simulink model "MotorControllerSimulation"  (R2016b)
settings: Solver=FixedStepAuto  StartTime=0.0  StopTime=20  FixedStep=Ts.controller  RelTol=1e-3
undefined symbols (not defined in the file): motor, sys_d, Ts
libraries: simulink x1
settings Model: Creator=Wall  LastModifiedBy=Wall

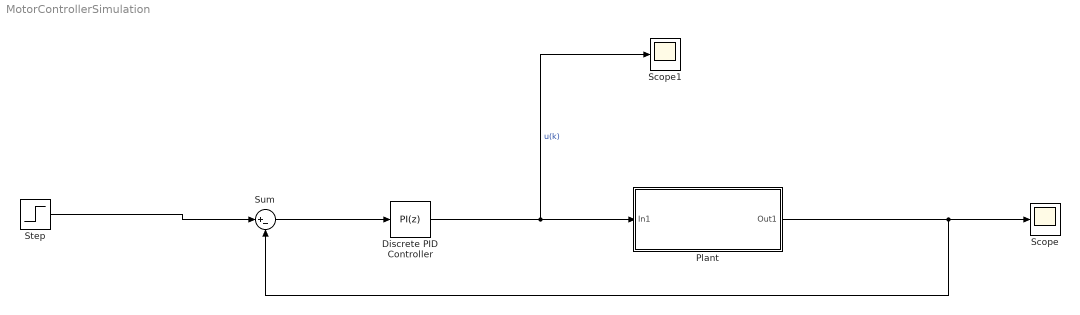
== system MotorControllerSimulation ==
  Discrete PID Controller : simulink/Continuous/PID Controller  Controller=PI  TimeDomain=Discrete-time  SampleTime=Ts.controller  IntegratorMethod=Forward Euler  FilterMethod=Forward Euler  Form=Parallel  UseFilter=off  ControllerParametersSource=internal  P=0.1  I=0.05  D=0  N=100  InitialConditionSource=internal  InitialConditionForIntegrator=0  InitialConditionForFilter=0  ExternalReset=none  LimitOutput=on  UpperSaturationLimit=motor.Imax  LowerSaturationLimit=-motor.Imax  LinearizeAsGain=off  AntiWindupMode=none  Kb=1  TrackingMode=off  Kt=1  PParamMin=[]  PParamMax=[]  IParamMin=[]  IParamMax=[]  DParamMin=[]  DParamMax=[]  NParamMin=[]  NParamMax=[]  KbParamMin=[]  KbParamMax=[]  KtParamMin=[]  KtParamMax=[]  POutMin=[]  POutMax=[]  IOutMin=[]  IOutMax=[]  DOutMin=[]  DOutMax=[]  NOutMin=[]  NOutMax=[]  KbOutMin=[]  KbOutMax=[]  KtOutMin=[]  KtOutMax=[]  IntegratorOutMin=[]  IntegratorOutMax=[]  FilterOutMin=[]  FilterOutMax=[]  SumOutMin=[]  SumOutMax=[]  SumI1OutMin=[]  SumI1OutMax=[]  SumI2OutMin=[]  SumI2OutMax=[]  SumI3OutMin=[]  SumI3OutMax=[]  SumDOutMin=[]  SumDOutMax=[]  SaturationOutMin=[]  SaturationOutMax=[]  IntegratorContinuousStateAttributes=''  IntegratorStateMustResolveToSignalObject=off  IntegratorRTWStateStorageClass=Auto  FilterContinuousStateAttributes=''  FilterStateMustResolveToSignalObject=off  FilterRTWStateStorageClass=Auto  DifferentiatorICPrevScaledInput=0  DifferentiatorOutMin=[]  DifferentiatorOutMax=[]
  Plant : Subsystem
  Scope : Scope
  Scope1 : Scope
  Step : Step  Time=2  After=200  SampleTime=Ts.controller
  Sum : Sum  Inputs=|+-
  wires:
  Discrete PID Controller/1 -> Plant/1(In1), Scope1/1  "u(k)"
  Sum/1 -> Discrete PID Controller/1
  Step/1 -> Sum/1
  Plant/1(Out1) -> Sum/2, Scope/1

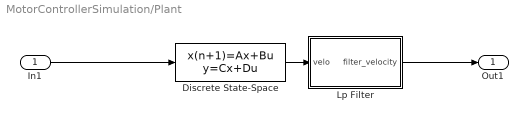
== system MotorControllerSimulation/Plant ==
  In1 : Inport
  Discrete State-Space : DiscreteStateSpace  A=sys_d.A  B=sys_d.B  C=sys_d.C  D=0  SampleTime=Ts.controller
  Lp Filter : MATLAB Function  TreatAsAtomicUnit=on
  Out1 : Outport
  wires:
  Lp Filter/1(filter_velocity) -> Out1/1
  In1/1 -> Discrete State-Space/1
  Discrete State-Space/1 -> Lp Filter/1(velo)

== matlab function MotorControllerSimulation/Plant/Lp Filter ==
  data: velo input; filter_velocity output; Ts parameter
function filter_velocity  = velocity(velo, Ts)

persistent f_velo;
persistent L_velo;


if isempty(f_velo)
   f_velo = 0;
   
   Tf_velo = 0.4;         % Time Constant % 0.04
   L_velo  = Ts.controller/(Tf_velo + Ts.controller);  % Filter gain
end

% LP Filter
f_velo = (1-L_velo) * f_velo + L_velo * velo;
filter_velocity = f_velo;
